simulink model "SendUdp2Kinarm_new"  (R2021b)
settings: Solver=FixedStepDiscrete  StartTime=0.0  StopTime=10  RelTol=1e-3  EnableMultiTasking=on
undefined symbols (not defined in the file or in its folder): f
libraries: instrumentlib x4
settings Model: Creator=The MathWorks, Inc.  LastModifiedBy=willy
settings SolverCC: AlgebraicLoopSolver=TrustRegion
settings DataIOCC: LimitDataPoints=on  SaveFormat=Array  ReturnWorkspaceOutputs=off
settings OptimizationCC: ExpressionDepthLimit=2147483647  InitFltsAndDblsToZero=on  LifeSpan=inf
settings DebuggingCC: UnderspecifiedInitializationDetection=Classic  MergeDetectMultiDrivingBlocksExec=none  SolverPrmCheckMsg=warning  FcnCallInpInsideContextMsg=warning  StateNameClashWarn=warning  SFUnexpectedBacktrackingDiag=warning  SFNoUnconditionalDefaultTransitionDiag=warning  SFExecutionAtInitializationDiag=none  SFMachineParentedDataDiag=warning  ArithmeticOperatorsInVariantConditions=warning
settings HardwareCC: ProdBitPerPointer=32  ProdBitPerSizeT=32  ProdBitPerPtrDiffT=32  ProdLargestAtomicFloat=None  ProdIntDivRoundTo=Undefined  ProdEndianess=Unspecified  ProdWordSize=32  ProdHWDeviceType=32-bit Generic
settings ModelReferenceCC: PropagateSignalLabelsOutOfModel=off
settings SFSimCC: SimUseLocalCustomCode=off  CustomCodeUndefinedFunction=UseInterfaceOnly
settings RTWCC: RTWUseLocalCustomCode=off
settings CodeAppCC: StateflowObjectComments=on
settings GRTTargetCC: TargetFcnLib=ansi_tfl_tmw_new.mat  TargetLangStandard=C89/C90 (ANSI)  CombineOutputUpdateFcns=off  GRTInterface=on
settings ConfigComp: CovScope=ReferencedModels  CovMetricSettings=dw  CovSaveCumulativeToWorkspaceVar=on  CovSaveSingleToWorkspaceVar=on  CovExternalEMLEnable=off

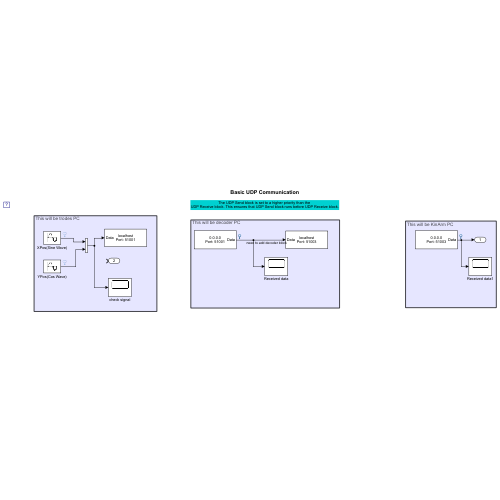
[thumbnail: Simulink's stored preview of the top-level diagram]
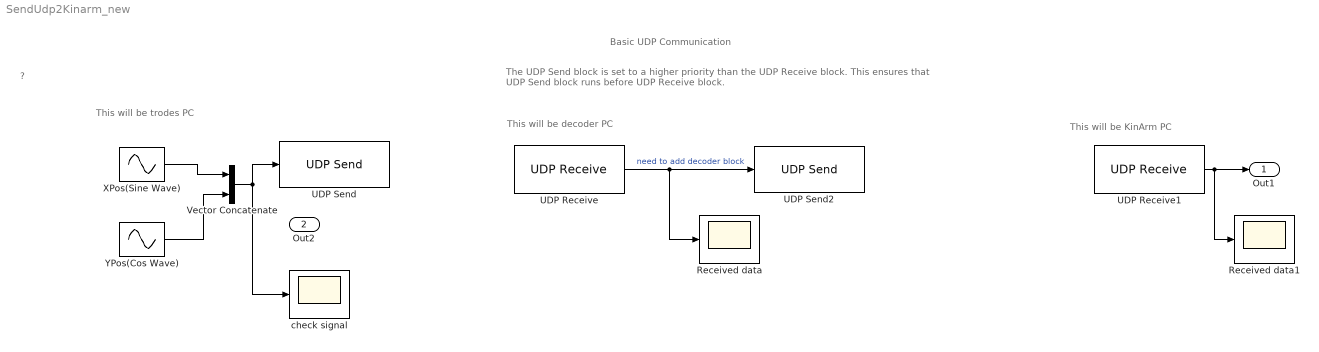
== system SendUdp2Kinarm_new ==
  note: This will be KinArm PC
  note: This will be trodes PC
  note: This will be decoder PC
  note: The UDP Send block is set to a higher priority than the
      | UDP Receive block. This ensures that UDP Send block runs before UDP Receive block.
  note: ?
  note: Basic UDP Communication
  Received data : Scope
      settings: Priority=4
  Received data1 : Scope
      settings: Priority=4
  UDP Receive : instrumentlib/UDP Receive  Priority=3  Host=localhost  Port=51000  LocalPort=51001  EnablePortSharing=off  GetLatestData=off  DataSize=[1 1]  DataType=double  ASCIIFormatting=%f,  Terminator=LF  ByteOrder=BigEndian  EnableBlockingMode=on  Timeout=5  SampleTime=0.1  LocalAddress=0.0.0.0
  UDP Receive1 : instrumentlib/UDP Receive  Priority=3  Host=localhost  Port=51002  LocalPort=51003  EnablePortSharing=on  GetLatestData=off  DataSize=[1 1]  DataType=double  ASCIIFormatting=%f,  Terminator=LF  ByteOrder=BigEndian  EnableBlockingMode=on  Timeout=5  SampleTime=0.1  LocalAddress=0.0.0.0
  UDP Send : instrumentlib/UDP Send  Priority=2  Host=localhost  Port=51001  LocalPort=51000  EnablePortSharing=off  ByteOrder=BigEndian  OutputDatagramPacketSize=512  EnableBlockingMode=on  LocalAddress=0.0.0.0
  UDP Send2 : instrumentlib/UDP Send  Priority=2  Host=localhost  Port=51003  LocalPort=51002  EnablePortSharing=on  ByteOrder=BigEndian  OutputDatagramPacketSize=512  EnableBlockingMode=on  LocalAddress=0.0.0.0
  Vector Concatenate : Concatenate  Mode=Multidimensional array  ConcatenateDimension=2
  XPos(Sine Wave) : Sin  Priority=1  SampleTime=0.1
  YPos(Cos Wave) : Sin  Priority=1  Phase=-pi/2  SampleTime=0.1
  check signal : Scope
      settings: Priority=4
  Out1 : Outport
  Out2 : Outport  Port=2
  wires:
  XPos(Sine Wave)/1 -> Vector Concatenate/1
  UDP Receive/1 -> UDP Send2/1, Received data/1  "need to add decoder block"
  YPos(Cos Wave)/1 -> Vector Concatenate/2
  Vector Concatenate/1 -> check signal/1, UDP Send/1
  UDP Receive1/1 -> Out1/1, Received data1/1
